simulink model "Houghline_real_nocolor_4"  (R2016a)
settings: Solver=FixedStepAuto  StartTime=0.0  StopTime=inf  RelTol=1e-3
undefined symbols (not defined in the file): gray, Rec, SDTV, strel
libraries: visionconversions x4, visiontextngfix x3, visiontransforms x3, visionfilter x2, dspvision x1, visionanalysis x1, visionstatistics x1, visionmorphops x1
settings Model: Creator=Yewly  LastModifiedBy=Yewly
settings GRTTargetCC: GeneratePreprocessorConditionals=Use local settings

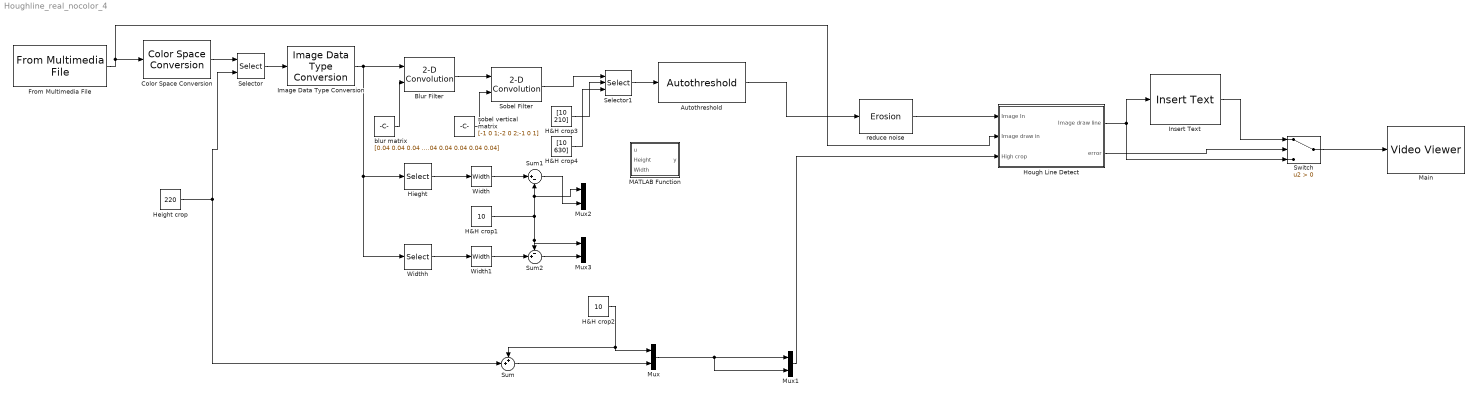
== system Houghline_real_nocolor_4 ==
  Autothreshold : visionconversions/Autothreshold  operator=>  threshOut=off  effMetricOut=off  userDefinedRange=off  umin=0  umax=255  outOfRngOpt=Warn and saturate  scaleThreshold=off  scaleFactor=1  P1Mode=Specify word length  P1WordLength=32  P1FracLength=30  P2Mode=Specify word length  P2WordLength=32  P2FracLength=22  P3Mode=Specify word length  P3WordLength=32  P3FracLength=14  P4Mode=Binary point scaling  P4WordLength=32  P4FracLength=15  Q1Mode=Specify word length  Q1WordLength=32  Q1FracLength=16  EMMode=Specify word length  EMWordLength=16  EMFracLength=14  roundingMode=Floor  overflowMode=off
  Blur Filter : visionfilter/2-D Convolution  outSize=Full  normalize=off  outputMode=Binary point scaling  outputWordLength=32  outputFracLength=12  prodOutputMode=Binary point scaling  prodOutputWordLength=32  prodOutputFracLength=10  roundingMode=Floor  overflowMode=off
  Color Space Conversion : visionconversions/Color Space  Conversion  conversion=Obsolete  conversionActive=R'G'B' to intensity  wp_str=D65  rec=Rec. 601 (SDTV)  sys=1125/60/2:1  imagePorts=One multidimensional signal
  From Multimedia File : dspvision/From Multimedia File  inputFilename=lane2.mp4  loop=on  numPlays=inf  outputStreams=Video only  videoDataType=single  audioDataType=int16  inheritSampleTime=on  userDefinedSampleTime=1/5  noAudioOutput=off  isIntensityVideo=off  fourcc=RGB  colorVideoFormat=One multidimensional signal  outputEOF=off  dataOrg=Column-major  audioFrameSize=1024  computeAudioFrameSize=off  outSamplingMode=Sample based
  H&H crop1 : Constant  Value=10  OutDataTypeStr=double
  H&H crop2 : Constant  Value=10  OutDataTypeStr=double
  H&H crop3 : Constant  Value=[10 210]  OutDataTypeStr=double
  H&H crop4 : Constant  Value=[10 630]  OutDataTypeStr=double
  Height crop : Constant  Value=220  OutDataTypeStr=double
  Hieght : Selector  NumberOfDimensions=2  InputPortWidth=3  IndexOptions=Select all,Index vector (dialog)  Indices=[1 3],1  OutputSizes=1,1
  "Hough Line Detect " : Subsystem
  Image Data Type Conversion : visionconversions/Image Data Type Conversion  outDT=double  isSigned=on  wordLen=16  numFracBits=0
  Insert Text : visiontextngfix/Insert Text  inputType=Obsolete  theText='ERROR'  getTextLocFrom=Specify via dialog  textLoc=[20 20]  getTextColorFrom=Specify via dialog  textColor=[255 0 0]  getTextIntensityFrom=Specify via dialog  textIntensity=0  getTextOpacityFrom=Specify via dialog  textOpacity=1.0  dummyVar2=0  dummyVar3=0  dummyVar4=0  imagePorts=One multidimensional signal  isInputTransposed=off  fontFace=LucidaSansRegular  dummyVar1=0  blockFontSize=32  antiAliased=on
  MATLAB Function : MATLAB Function  TreatAsAtomicUnit=on
  Main : VideoViewer  colormapValue=gray(256)  FigPos=[7.4 550 544 444.8]
  Mux{,1..3} (4 alike) : Mux  Inputs=2
      Mux2 settings: DisplayOption=signals
      Mux3 settings: DisplayOption=signals
  Selector : Selector  NumberOfDimensions=2  InputPortWidth=3  IndexOptions=Starting index (port),Select all  Indices=220,1  OutputSizes=220,1
  Selector1 : Selector  NumberOfDimensions=2  InputPortWidth=3  IndexOptions=Starting and ending indices (port),Starting and ending indices (port)  Indices=10,10  OutputSizes=210,630
  Sobel Filter : visionfilter/2-D Convolution  outSize=Full  normalize=off  outputMode=Binary point scaling  outputWordLength=32  outputFracLength=12  prodOutputMode=Binary point scaling  prodOutputWordLength=32  prodOutputFracLength=10  roundingMode=Floor  overflowMode=off
  Sum : Sum  Inputs=++|
  Sum1 : Sum  Inputs=|+-
  Sum2 : Sum  Inputs=-+|
  Switch : Switch  Criteria=u2 > Threshold
  Width : Width
  Width1 : Width
  "Widthh " : Selector  NumberOfDimensions=2  InputPortWidth=3  IndexOptions=Index vector (dialog),Select all  Indices=1,2  OutputSizes=1,1
  blur matrix : Constant  Value=[0.04 0.04 0.04 0.04 0.04;0.04 0.04 0.04 0.04 0.04;0.04 0.04 0.04 0.04 0.04;0.04 0.04 0.04 0.04 0.04;0.04 0.04 0.04 0.04 0.04]  OutDataTypeStr=double
  "reduce noise " : visionmorphops/Erosion  nhoodsrc=Specify via dialog  strel=strel('square',2)
  sobel vertical matrix : Constant  Value=[-1 0 1;-2 0 2;-1 0 1]  OutDataTypeStr=double
  wires:
  From Multimedia File/1 -> "Hough Line Detect "/2("Image draw in "), Color Space Conversion/1
  Selector/1 -> Image Data Type Conversion/1
  Sobel Filter/1 -> Selector1/1
  Blur Filter/1 -> Sobel Filter/1
  Selector1/1 -> Autothreshold/1
  Image Data Type Conversion/1 -> Blur Filter/1, "Widthh "/1, Hieght/1
  blur matrix/1 -> Blur Filter/2
  sobel vertical matrix/1 -> Sobel Filter/2
  Height crop/1 -> Selector/2, Sum/2
  Mux/1 -> Mux1/2, Mux1/1
  Mux1/1 -> "Hough Line Detect "/3(High crop)
  Sum/1 -> Mux/2
  Switch/1 -> Main/1
  "Hough Line Detect "/2(error) -> Switch/2
  "Hough Line Detect "/1("Image draw line ") -> Insert Text/1, Switch/3
  Insert Text/1 -> Switch/1
  Autothreshold/1 -> "reduce noise "/1
  "reduce noise "/1 -> "Hough Line Detect "/1(Image In)
  Color Space Conversion/1 -> Selector/1
  "Widthh "/1 -> Width1/1
  Hieght/1 -> Width/1
  Width/1 -> Sum1/1
  Width1/1 -> Sum2/2
  H&H crop1/1 -> Sum1/2, Mux2/1, Mux3/1, Sum2/1
  Sum1/1 -> Mux2/2
  Sum2/1 -> Mux3/2
  H&H crop2/1 -> Mux/1, Sum/1
  H&H crop3/1 -> Selector1/2
  H&H crop4/1 -> Selector1/3

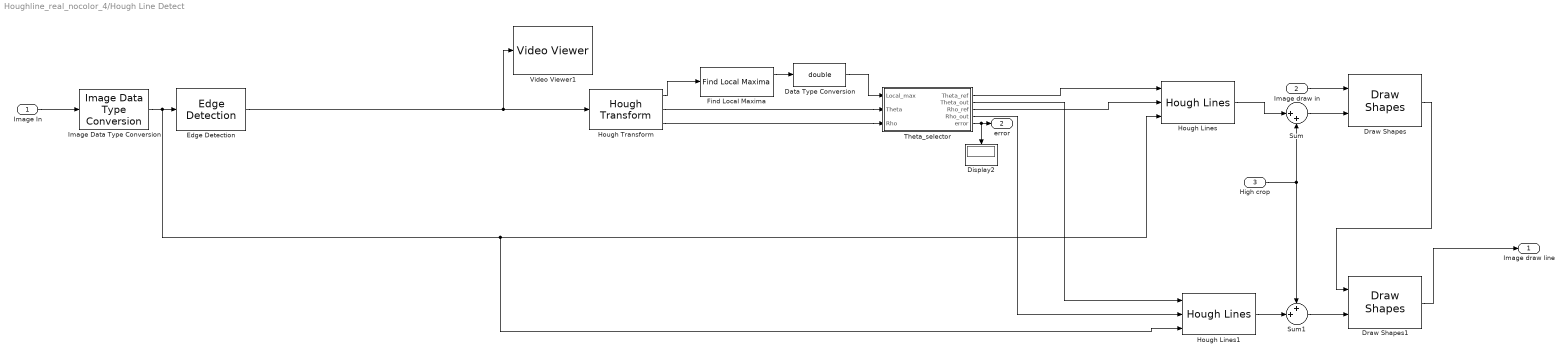
== system Houghline_real_nocolor_4/Hough Line Detect  ==
  Image In : Inport
  "Image draw in " : Inport  Port=2
  High crop : Inport  Port=3
  Data Type Conversion : DataTypeConversion  OutDataTypeStr=double
  Display2 : Display
  Draw Shapes : visiontextngfix/Draw Shapes  shape=Lines  fill=off  lineWidth=10  fillClrSource=Specify via dialog  display=User-specified value  intensity=200  color=[0 255 0]  opacity=0.6  viewport=Entire image  antialiasing=off  inType=Obsolete  imagePorts=One multidimensional signal  prodOutputMode=Binary point scaling  prodOutputWordLength=32  prodOutputFracLength=14  memoryMode=Specify word length  memoryWordLength=16  memoryFracLength=14  roundingMode=Floor  overflowMode=off
  Draw Shapes1 : visiontextngfix/Draw Shapes  shape=Lines  fill=off  lineWidth=10  fillClrSource=Specify via dialog  display=User-specified value  intensity=200  color=[0 0 255]  opacity=0.6  viewport=Entire image  antialiasing=off  inType=Obsolete  imagePorts=One multidimensional signal  prodOutputMode=Binary point scaling  prodOutputWordLength=32  prodOutputFracLength=14  memoryMode=Specify word length  memoryWordLength=16  memoryFracLength=14  roundingMode=Floor  overflowMode=off
  Edge Detection : visionanalysis/Edge Detection  method=Sobel  outputType=Binary image  userDefinedThreshold=off  thresholdSource=Specify via dialog  threshold=20  thresholdTuning=2  edgeThinning=off  threshold_canny=[0.25 0.60]  autoPercent=70  sigma=1  prodOutputMode=Binary point scaling  prodOutputWordLength=32  prodOutputFracLength=8  roundingMode=Floor  overflowMode=off
  Find Local Maxima : visionstatistics/Find Local Maxima  num_peaks=15  nhood_size=[5 7]  src_thresh=Obsolete9b  src_thresh_inuse=Specify via dialog  threshold=10  inputIsHough=on  dt_peak=uint32  isOutVarDim=off  dt_count=uint32
  Hough Lines : visiontransforms/Hough Lines  sineCompMethod=Trigonometric function  thetaRes=pi/180  firstCoeffMode=Specify word length  firstCoeffWordLength=16  firstCoeffFracLength=15  prodOutputMode=Binary point scaling  prodOutputWordLength=32  prodOutputFracLength=16  roundingMode=Nearest  overflowMode=on
  Hough Lines1 : visiontransforms/Hough Lines  sineCompMethod=Trigonometric function  thetaRes=pi/180  firstCoeffMode=Specify word length  firstCoeffWordLength=16  firstCoeffFracLength=15  prodOutputMode=Binary point scaling  prodOutputWordLength=32  prodOutputFracLength=16  roundingMode=Nearest  overflowMode=on
  Hough Transform : visiontransforms/Hough Transform  theta_res=pi/360  rho_res=1  out_theta_rho=on  outdtmode=double  firstCoeffMode=Binary point scaling  firstCoeffWordLength=16  firstCoeffFracLength=14  secondCoeffMode=Binary point scaling  secondCoeffWordLength=32  secondCoeffFracLength=16  outputMode=Binary point scaling  outputWordLength=16  outputFracLength=0  accumMode=Binary point scaling  accumWordLength=32  accumFracLength=20  prodOutputMode=Binary point scaling  prodOutputWordLength=32  prodOutputFracLength=20  memoryMode=Binary point scaling  memoryWordLength=32  memoryFracLength=16  roundingMode=Nearest  overflowMode=on
  Image Data Type Conversion : visionconversions/Image Data Type Conversion  outDT=double  isSigned=on  wordLen=16  numFracBits=0
  Sum : Sum  Inputs=|++
  Sum1 : Sum  Inputs=++|
  Theta_selector : MATLAB Function  TreatAsAtomicUnit=on
  Video Viewer1 : VideoViewer  colormapValue=gray(256)  FigPos=[14.6 810 541.6 205.6]
  "Image draw line " : Outport
  error : Outport  Port=2
  wires:
  Draw Shapes1/1 -> "Image draw line "/1
  Hough Transform/1 -> Find Local Maxima/1
  Draw Shapes/1 -> Draw Shapes1/1
  Image Data Type Conversion/1 -> Hough Lines1/3, Hough Lines/3, Edge Detection/1
  Image In/1 -> Image Data Type Conversion/1
  "Image draw in "/1 -> Draw Shapes/1
  Hough Lines/1 -> Sum/1
  Sum/1 -> Draw Shapes/2
  High crop/1 -> Sum/2, Sum1/1
  Sum1/1 -> Draw Shapes1/2
  Hough Lines1/1 -> Sum1/2
  Find Local Maxima/1 -> Data Type Conversion/1
  Data Type Conversion/1 -> Theta_selector/1(Local_max)
  Hough Transform/2 -> Theta_selector/2(Theta)
  Hough Transform/3 -> Theta_selector/3(Rho)
  Theta_selector/1(Theta_ref) -> Hough Lines/1
  Theta_selector/3(Rho_ref) -> Hough Lines/2
  Theta_selector/2(Theta_out) -> Hough Lines1/1
  Theta_selector/4(Rho_out) -> Hough Lines1/2
  Theta_selector/5(error) -> error/1, Display2/1
  Edge Detection/1 -> Hough Transform/1, Video Viewer1/1

== matlab function Houghline_real_nocolor_4/MATLAB Function ==
  data: u input; y output; Height input; Width input
function y = fcn(u,Height,Width)
%#codegen
y = u(Height(1):Height(2),Width(1),Width(2));

== matlab function Houghline_real_nocolor_4/Hough Line Detect /Theta_selector ==
  data: Theta_ref output; Theta_out output; Rho_ref output; Local_max input; Theta input; Rho input; Rho_out output; error output
function [Theta_ref,Theta_out,Rho_ref,Rho_out,error] = Theta_selector(Local_max,Theta,Rho)
[H,W] = size(Local_max);
mem = 100;
idx_out = 1;
error = 0;
for x = 1:H
if Theta(Local_max(x,1)) > 0
    Theta_ref = Theta(Local_max(x,1));
    if Theta_ref > 1
        error = 1;
    end
    Rho_ref = Rho(Local_max(x,2));
    break;
else
    Theta_ref=Theta(Local_max(x,1));
    Rho_ref = Rho(Local_max(x,2));
end
end

for x = 1:H
A = abs(Theta(Local_max(x,1)) + Theta_ref);
if A < mem
    mem = A;
    idx_out = x;
end
end
Theta_out = Theta(Local_max(idx_out,1));
if Theta_out > 1 
        error = 1;
end
if (Theta_out > 0 && Theta_ref > 0) | (Theta_out < 0 && Theta_ref < 0)
        error = 1;
end
Rho_out = Rho(Local_max(idx_out,2));
